simulink library "AircraftModel"  (R2016b)
settings: Solver=VariableStepAuto  StartTime=0.0  StopTime=10.0  RelTol=1e-3
values from neighbouring files (symbols this model uses):
  AC = miniMUTT_config    [UAV_config.m]
undefined symbols (not defined in the file or in its folder): Env, m, s
undefined symbols (not defined in the file): TrimCondition
libraries: aerolib6dofsys x4, Environment_Lib x2, aerolibconvert2 x2, aerolibatmos2 x1, aerolibgravity2 x1, aerolibutil x1, AuxEq_Lib x1, aerolibadyn x1, Gravity_Lib x1, Propulsion_Lib x1
settings Model: Creator=UAVLAB  LastModifiedBy=UAVLAB

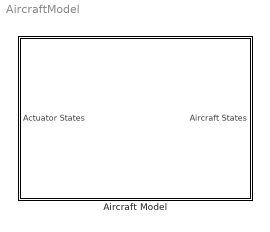
== system AircraftModel ==
  Aircraft Model : Subsystem

== system AircraftModel/Aircraft Model ==
  Actuator States : Inport  OutDataTypeStr=Bus: Actuators
  Bus Creator : BusCreator  Inputs=3  OutDataTypeStr=Bus: States
      settings: InheritFromInputs=off
  Environment Model : Subsystem
  Nonlinear UAV Model : Subsystem
  Aircraft States : Outport  OutDataTypeStr=Bus: States
  wires:
  Bus Creator/1 -> Aircraft States/1
  Environment Model/1(EnvData) -> Bus Creator/1, Nonlinear UAV Model/1(EnvData)  "EnvData"
  Nonlinear UAV Model/2(AuxVar) -> Environment Model/2(AuxVar), Bus Creator/2  "AuxVar"
  Nonlinear UAV Model/1(RigidStates) -> Bus Creator/3, Environment Model/1(RigidStates)  "RigidStates"
  Actuator States/1 -> Nonlinear UAV Model/2(Actuator States)

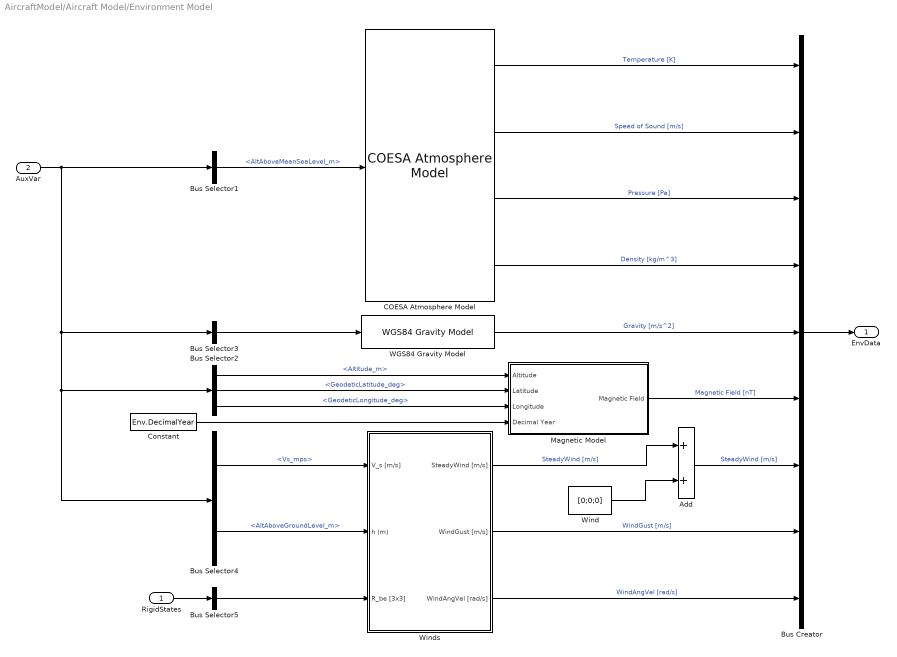
== system AircraftModel/Aircraft Model/Environment Model ==
  RigidStates : Inport  OutDataTypeStr=Bus: RigidStates
  AuxVar : Inport  Port=2  OutDataTypeStr=Bus: AuxVar
  Add : Sum
  Bus Creator : BusCreator  Inputs=9  OutDataTypeStr=Bus: EnvData
      settings: InheritFromInputs=off
  Bus Selector1 : BusSelector  OutputSignals=Nav.AltAboveMeanSeaLevel_m
  Bus Selector2 : BusSelector  OutputSignals=Nav.Altitude_m,Nav.GeodeticLatitude_deg,Nav.GeodeticLongitude_deg
  Bus Selector3 : BusSelector  OutputSignals=Nav.GeodeticLatitude_deg,Nav.GeodeticLongitude_deg,Nav.Altitude_m  OutputAsBus=on
  Bus Selector4 : BusSelector  OutputSignals=WindAxesParams.Vs_mps,Nav.AltAboveGroundLevel_m
  Bus Selector5 : BusSelector  OutputSignals=DCM  OutputAsBus=on
  COESA Atmosphere Model : aerolibatmos2/COESA Atmosphere Model  units=Metric (MKS)  spec=1976 COESA-extended U.S. Standard Atmosphere  model=Profile  profile_var=High temperature  profile_percent=1%  profile_alt=5 km (16404 ft)  envelope_var=High temperature  envelope_percent=1%  action=Warning
  Constant : Constant  Value=Env.DecimalYear
  Magnetic Model : Subsystem  BlockChoice=WMM Bypass
      settings: AttributesFormatString=%<BlockChoice>  TemplateBlock=Environment_Lib/Magnetic Model  MemberBlocks=WMM 2005,WMM Bypass
  "WGS84 Gravity Model " : aerolibgravity2/WGS84 Gravity Model   model=WGS84 Taylor Series  units=Metric (MKS)  no_atmos=on  precessing=on  jd_loc=off  month=October  day=10  year=2004  no_centrifugal=on  action=Warning
  Wind : Constant  Value=[0;0;0]
  Winds : Subsystem  BlockChoice=Wind Bypass
      settings: AttributesFormatString=%<BlockChoice>  TemplateBlock=Environment_Lib/Winds  MemberBlocks=Wind & Turbulence,Wind Bypass
  EnvData : Outport  OutDataTypeStr=Bus: EnvData
  wires:
  Winds/1(SteadyWind [m/s]) -> Add/1  "SteadyWind [m/s]"
  Wind/1 -> Add/2
  Winds/3(WindAngVel [rad/s]) -> Bus Creator/9  "WindAngVel [rad/s]"
  Winds/2(WindGust [m/s]) -> Bus Creator/8  "WindGust [m/s]"
  Add/1 -> Bus Creator/7  "SteadyWind [m/s]"
  Magnetic Model/1(Magnetic Field) -> Bus Creator/6  "Magnetic Field [nT]"
  "WGS84 Gravity Model "/1 -> Bus Creator/5  "Gravity [m/s^2]"
  Bus Selector5/1 -> Winds/3(R_be [3x3])
  RigidStates/1 -> Bus Selector5/1
  AuxVar/1 -> Bus Selector1/1, Bus Selector2/1, Bus Selector4/1, Bus Selector3/1
  Constant/1 -> Magnetic Model/4(Decimal Year)
  Bus Selector3/1 -> "WGS84 Gravity Model "/1
  Bus Selector2/3 -> Magnetic Model/3(Longitude)  "<GeodeticLongitude_deg>"
  Bus Selector2/2 -> Magnetic Model/2(Latitude)  "<GeodeticLatitude_deg>"
  Bus Selector2/1 -> Magnetic Model/1(Altitude)  "<Altitude_m>"
  COESA Atmosphere Model/4 -> Bus Creator/4  "Density [kg/m^3]"
  COESA Atmosphere Model/1 -> Bus Creator/1  "Temperature [K]"
  COESA Atmosphere Model/2 -> Bus Creator/2  "Speed of Sound [m/s]"
  COESA Atmosphere Model/3 -> Bus Creator/3  "Pressure [Pa]"
  Bus Selector1/1 -> COESA Atmosphere Model/1  "<AltAboveMeanSeaLevel_m>"
  Bus Creator/1 -> EnvData/1
  Bus Selector4/1 -> Winds/1(V_s [m/s])  "<Vs_mps>"
  Bus Selector4/2 -> Winds/2(h (m))  "<AltAboveGroundLevel_m>"

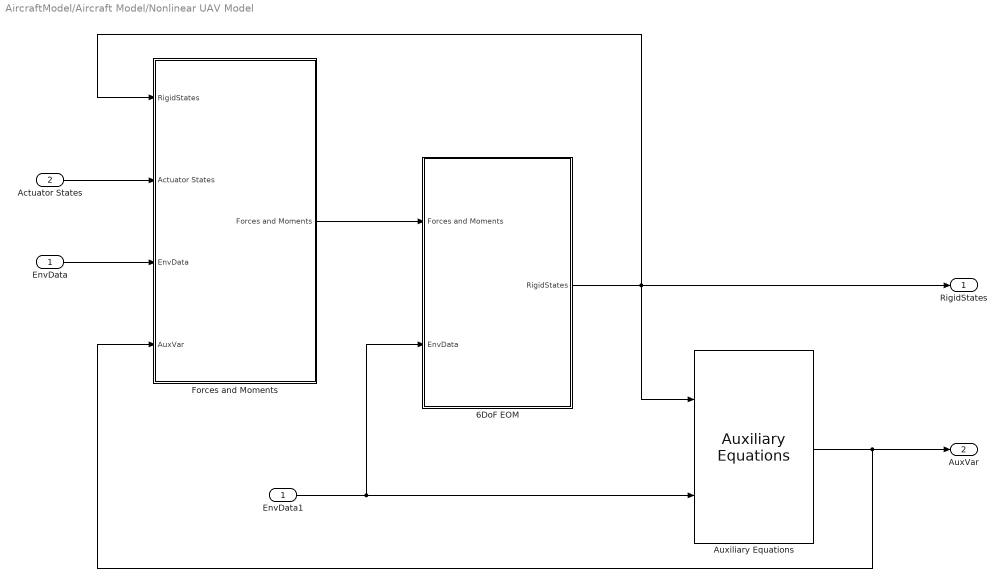
== system AircraftModel/Aircraft Model/Nonlinear UAV Model ==
  EnvData : Inport  OutDataTypeStr=Bus: EnvData
  Actuator States : Inport  Port=2  OutDataTypeStr=Bus: Actuators
  6DoF EOM : Subsystem  mask(6DoF EoM (Body Axis)){units=Metric (MKS), mtype=Fixed, rep=Euler Angles, xme_0=TrimCondition.InertialIni, Vm_0=TrimCondition.VelocitiesIni, eul_0=TrimCondition.AttitudeIni, pm_0=TrimCondition.RatesIni, mass_0=AC.Mass, mass_e=0.5, mass_f=2.0, inertia=AC.Inertia.Matrix, inertia_e=eye(3), inertia_f=2*eye(3), k_quat=1.0}
      mask prompts: mtype "Mass type:"; rep "Representation:"; xme_0 "Initial position in inertial axes [Xe,Ye,Ze]:"; Vm_0 "Initial velocity in body axes [U,v,w]:"; eul_0 "Initial Euler orientation [roll, pitch, yaw]:"; pm_0 "Initial body rotation rates [p,q,r]:"; mass_0 "Initial mass:"; mass_e "Empty mass:"; mass_f "Full mass:"; inertia_e "Empty inertia matrix:"; inertia_f "Full inertia matrix:"; k_quat "Gain for quaternion normalization:"
      mask help:
      | Integrate the six-degrees-of-freedom equations of motion in body axis.
      |
      | This block has been modified from the original Aerospace Blockset
      | implementation. The inertial position vector (Xe) is no longer computed.
      | The original block did not have a way to add steady state winds to the
      | inertial velocities (Ve) prior to integrating to get Xe. Therefore, this
      | step is performed in the Auxiliary Equations block.
      mask Help: eval('asbhelp(''sixdof_euler_angles'')');
      mask TypeOptions units: Metric (MKS) | English (Velocity in ft/s) | English (Velocity in kts)
      mask TypeOptions mtype: Fixed | Simple Variable | Custom Variable
      mask Callback mtype: aeroicon('aeroblk6dofbody');
      mask TypeOptions rep: Euler Angles | Quaternion
      mask Callback rep: aeroicon('aeroblk6dofbody');
  Auxiliary Equations : AuxEq_Lib/Auxiliary Equations
  EnvData1 : InportShadow  OutDataTypeStr=Bus: EnvData
  Forces and Moments : Subsystem
  RigidStates : Outport  OutDataTypeStr=Bus: RigidStates
  AuxVar : Outport  Port=2  OutDataTypeStr=Bus: AuxVar
  wires:
  Auxiliary Equations/1 -> AuxVar/1, Forces and Moments/4(AuxVar)
  6DoF EOM/1(RigidStates) -> Auxiliary Equations/1, RigidStates/1, Forces and Moments/1(RigidStates)
  EnvData1/1 -> Auxiliary Equations/2, 6DoF EOM/2(EnvData)
  EnvData/1 -> Forces and Moments/3(EnvData)
  Actuator States/1 -> Forces and Moments/2(Actuator States)
  Forces and Moments/1(Forces and Moments) -> 6DoF EOM/1(Forces and Moments)

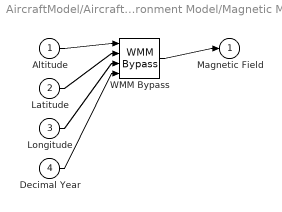
== system AircraftModel/Aircraft Model/Environment Model/Magnetic Model ==
  Altitude : Inport
  Latitude : Inport  Port=2
  Longitude : Inport  Port=3
  Decimal Year : Inport  Port=4
  WMM Bypass : Environment_Lib/WMM Bypass  units=Metric (MKS)  time_in=on  month=August  day=1  year=2009  action=None  h_out=off  dec_out=off  inc_out=off  ti_out=off
  Magnetic Field : Outport
  wires:
  WMM Bypass/1 -> Magnetic Field/1
  Decimal Year/1 -> WMM Bypass/4
  Longitude/1 -> WMM Bypass/3
  Latitude/1 -> WMM Bypass/2
  Altitude/1 -> WMM Bypass/1

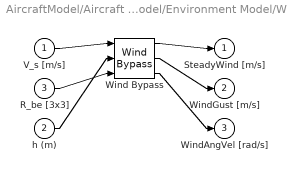
== system AircraftModel/Aircraft Model/Environment Model/Winds ==
  V_s [m/s] : Inport
  h (m) : Inport  Port=2
  R_be [3x3] : Inport  Port=3
  Wind Bypass : Environment_Lib/Wind Bypass
  SteadyWind [m/s] : Outport
  WindGust [m/s] : Outport  Port=2
  WindAngVel [rad/s] : Outport  Port=3
  wires:
  Wind Bypass/3 -> WindAngVel [rad/s]/1
  Wind Bypass/2 -> WindGust [m/s]/1
  Wind Bypass/1 -> SteadyWind [m/s]/1
  R_be [3x3]/1 -> Wind Bypass/3
  h (m)/1 -> Wind Bypass/2
  V_s [m/s]/1 -> Wind Bypass/1

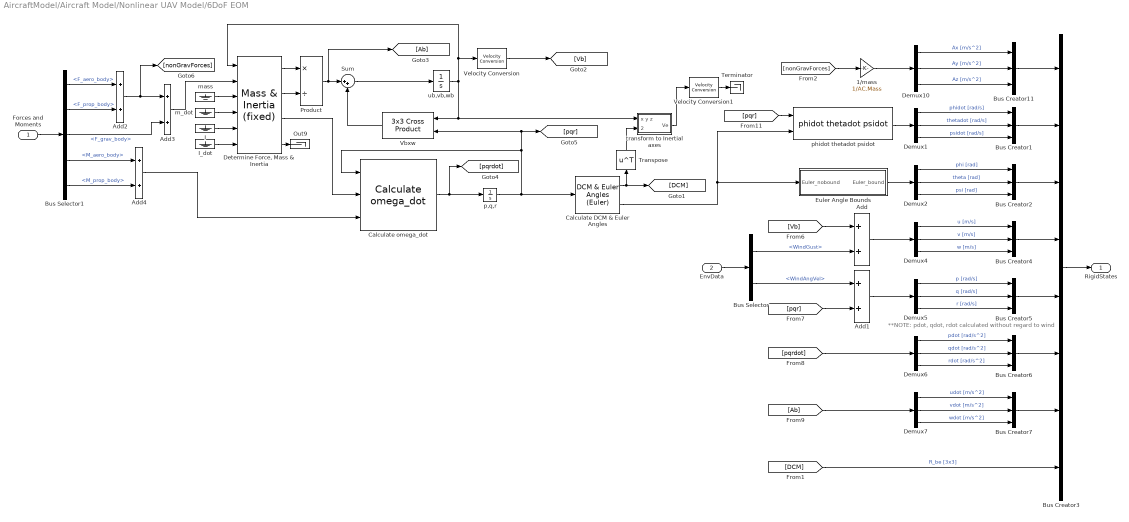
== system AircraftModel/Aircraft Model/Nonlinear UAV Model/6DoF EOM ==
  note: **NOTE: pdot, qdot, rdot calculated without regard to wind
  Forces and Moments : Inport
  EnvData : Inport  Port=2  OutDataTypeStr=Bus: EnvData
  1/mass : Gain  Gain=1/AC.Mass
  Add{,1..4} (5 alike) : Sum
  Bus Creator{1..2,4..7,11} (7 alike) : BusCreator  Inputs=3
  Bus Selector : BusSelector  OutputSignals=WindGust,WindAngVel
  Bus Selector1 : BusSelector  OutputSignals=AeroLoads.F_aero_body,F_prop_body,F_grav_body,AeroLoads.M_aero_body,M_prop_body
  Bus Creator3 : BusCreator  Inputs=8  OutDataTypeStr=Bus: RigidStates
      settings: InheritFromInputs=off
  Calculate DCM & Euler Angles : aerolib6dofsys/DCM & Euler Angles (Euler)  SystemSampleTime=-1
  Calculate omega_dot : aerolib6dofsys/Calculate omega_dot  SystemSampleTime=-1
  Demux{1..2,4..7,10} (7 alike) : Demux  Outputs=3
  "Determine Force, Mass & Inertia" : aerolib6dofsys/Mass & Inertia (fixed)  SystemSampleTime=-1
  Euler Angle Bounds : Subsystem
  I : Ground
  I_dot : Ground
  Out9 : Terminator
  Product : Product  Inputs=*/  SaturateOnIntegerOverflow=on  OutDataTypeStr=Inherit: Same as first input
  Sum : Sum  Inputs=|++  SaturateOnIntegerOverflow=on
  Terminator : Terminator
  Transpose : Math  Operator=transpose  SaturateOnIntegerOverflow=on
  Vbxw : aerolibutil/3x3 Cross Product
  Velocity Conversion : aerolibconvert2/Velocity Conversion  IU=m/s  OU=m/s
  Velocity Conversion1 : aerolibconvert2/Velocity Conversion  IU=m/s  OU=m/s
  m_dot : Ground
  mass : Ground
  "p,q,r " : Integrator  InitialCondition=pm_0
  phidot thetadot psidot : aerolib6dofsys/DCM & Euler Angles (Euler)/phidot thetadot psidot
  "transform to Inertial axes " : Subsystem  mask(Vector Transformation){}
      mask Display: disp('L_EB')
  ub,vb,wb : Integrator  InitialCondition=convvel(Vm_0,'m/s','m/s')
  RigidStates : Outport  OutDataTypeStr=Bus: RigidStates
  wires:
  [DCM] -> Bus Creator3/8  "R_be [3x3]"
  Bus Creator11/1 -> Bus Creator3/1
  Bus Creator2/1 -> Bus Creator3/3
  Bus Creator1/1 -> Bus Creator3/2
  Bus Creator7/1 -> Bus Creator3/7
  Bus Creator6/1 -> Bus Creator3/6
  Bus Creator5/1 -> Bus Creator3/5
  Bus Creator4/1 -> Bus Creator3/4
  Bus Creator3/1 -> RigidStates/1
  Add4/1 -> Calculate omega_dot/3
  Bus Selector1/5 -> Add4/2  "<M_prop_body>"
  Bus Selector1/4 -> Add4/1  "<M_aero_body>"
  Add3/1 -> "Determine Force, Mass & Inertia"/2
  Bus Selector1/3 -> Add3/2  "<F_grav_body>"
  Add2/1 -> Add3/1, [nonGravForces]
  Bus Selector1/2 -> Add2/2  "<F_prop_body>"
  Bus Selector1/1 -> Add2/1  "<F_aero_body>"
  Forces and Moments/1 -> Bus Selector1/1
  Demux10/3 -> Bus Creator11/3  "Az [m/s^2]"
  Demux10/2 -> Bus Creator11/2  "Ay [m/s^2]"
  Demux10/1 -> Bus Creator11/1  "Ax [m/s^2]"
  1/mass/1 -> Demux10/1
  [nonGravForces] -> 1/mass/1
  Euler Angle Bounds/1(Euler_bound) -> Demux2/1
  Demux2/1 -> Bus Creator2/1  "phi [rad]"
  Demux2/2 -> Bus Creator2/2  "theta [rad]"
  Demux2/3 -> Bus Creator2/3  "psi [rad]"
  Calculate DCM & Euler Angles/2 -> phidot thetadot psidot/2, Euler Angle Bounds/1(Euler_nobound)
  [pqr] -> phidot thetadot psidot/1
  phidot thetadot psidot/1 -> Demux1/1
  Demux1/1 -> Bus Creator1/1  "phidot [rad/s]"
  Demux1/2 -> Bus Creator1/2  "thetadot [rad/s]"
  Demux1/3 -> Bus Creator1/3  "psidot [rad/s]"
  Demux7/1 -> Bus Creator7/1  "udot [m/s^2]"
  Demux7/2 -> Bus Creator7/2  "vdot [m/s^2]"
  Demux7/3 -> Bus Creator7/3  "wdot [m/s^2]"
  [Ab] -> Demux7/1
  Demux6/1 -> Bus Creator6/1  "pdot [rad/s^2]"
  Demux6/2 -> Bus Creator6/2  "qdot [rad/s^2]"
  Demux6/3 -> Bus Creator6/3  "rdot [rad/s^2]"
  [pqrdot] -> Demux6/1
  Add1/1 -> Demux5/1
  Demux5/1 -> Bus Creator5/1  "p [rad/s]"
  Demux5/2 -> Bus Creator5/2  "q [rad/s]"
  Demux5/3 -> Bus Creator5/3  "r [rad/s]"
  [pqr] -> Add1/2
  Demux4/1 -> Bus Creator4/1  "u [m/s]"
  Demux4/2 -> Bus Creator4/2  "v [m/s]"
  Demux4/3 -> Bus Creator4/3  "w [m/s]"
  Add/1 -> Demux4/1
  [Vb] -> Add/1
  Bus Selector/2 -> Add1/1  "<WindAngVel>"
  Bus Selector/1 -> Add/2  "<WindGust>"
  EnvData/1 -> Bus Selector/1
  Velocity Conversion1/1 -> Terminator/1
  Velocity Conversion/1 -> [Vb]
  "Determine Force, Mass & Inertia"/3 -> Calculate omega_dot/2
  Vbxw/1 -> Sum/2
  ub,vb,wb/1 -> "transform to Inertial axes "/1(x y z), Vbxw/1, Velocity Conversion/1, "Determine Force, Mass & Inertia"/1
  Sum/1 -> ub,vb,wb/1
  "transform to Inertial axes "/1(Ve) -> Velocity Conversion1/1
  "p,q,r "/1 -> Calculate DCM & Euler Angles/1, Vbxw/2, [pqr], Calculate omega_dot/1
  Product/1 -> Sum/1, [Ab]
  Calculate DCM & Euler Angles/1 -> Transpose/1, [DCM]
  Transpose/1 -> "transform to Inertial axes "/2(transform coefficients)
  mass/1 -> "Determine Force, Mass & Inertia"/3
  "Determine Force, Mass & Inertia"/2 -> Product/2
  m_dot/1 -> "Determine Force, Mass & Inertia"/4
  "Determine Force, Mass & Inertia"/4 -> Out9/1
  Calculate omega_dot/1 -> "p,q,r "/1, [pqrdot]
  I/1 -> "Determine Force, Mass & Inertia"/5
  I_dot/1 -> "Determine Force, Mass & Inertia"/6
  "Determine Force, Mass & Inertia"/1 -> Product/1

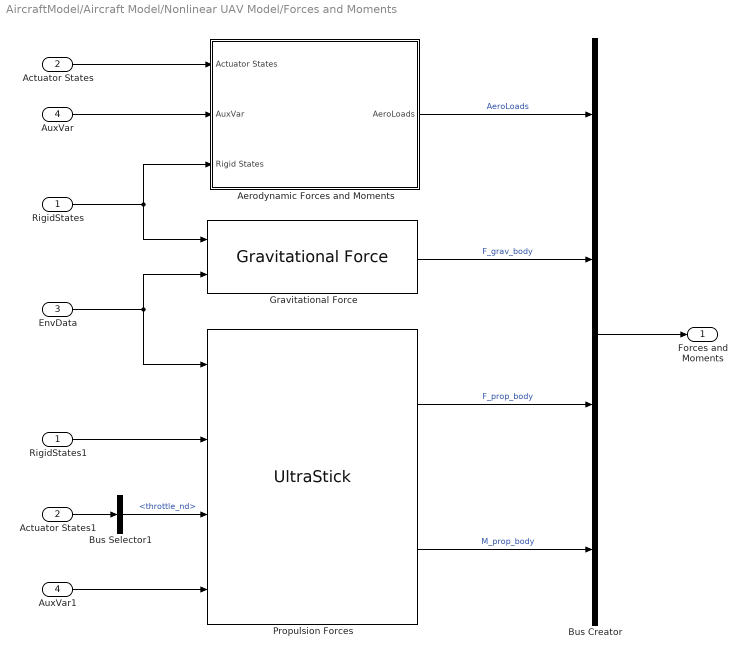
== system AircraftModel/Aircraft Model/Nonlinear UAV Model/Forces and Moments ==
  RigidStates : Inport  OutDataTypeStr=Bus: RigidStates
  Actuator States : Inport  Port=2  OutDataTypeStr=Bus: Actuators
  EnvData : Inport  Port=3  OutDataTypeStr=Bus: EnvData
  AuxVar : Inport  Port=4  OutDataTypeStr=Bus: AuxVar
  Actuator States1 : InportShadow  Port=2  OutDataTypeStr=Bus: Actuators
  Aerodynamic Forces and Moments : Subsystem
  AuxVar1 : InportShadow  Port=4  OutDataTypeStr=Bus: AuxVar
  Bus Selector1 : BusSelector  OutputSignals=throttle_nd
  Bus Creator : BusCreator  Inputs=4
  "Gravitational Force " : Gravity_Lib/Gravitational Force 
  Propulsion Forces : Propulsion_Lib/UltraStick
  RigidStates1 : InportShadow  OutDataTypeStr=Bus: RigidStates
  Forces and Moments : Outport
  wires:
  AuxVar1/1 -> Propulsion Forces/4
  RigidStates/1 -> Aerodynamic Forces and Moments/3(Rigid States), "Gravitational Force "/1
  AuxVar/1 -> Aerodynamic Forces and Moments/2(AuxVar)
  Bus Creator/1 -> Forces and Moments/1
  Propulsion Forces/2 -> Bus Creator/4  "M_prop_body"
  Propulsion Forces/1 -> Bus Creator/3  "F_prop_body"
  "Gravitational Force "/1 -> Bus Creator/2  "F_grav_body"
  RigidStates1/1 -> Propulsion Forces/2
  Aerodynamic Forces and Moments/1(AeroLoads) -> Bus Creator/1  "AeroLoads"
  Bus Selector1/1 -> Propulsion Forces/3  "<throttle_nd>"
  EnvData/1 -> "Gravitational Force "/2, Propulsion Forces/1
  Actuator States1/1 -> Bus Selector1/1
  Actuator States/1 -> Aerodynamic Forces and Moments/1(Actuator States)

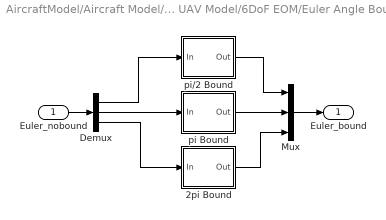
== system AircraftModel/Aircraft Model/Nonlinear UAV Model/6DoF EOM/Euler Angle Bounds ==
  Euler_nobound : Inport
  2pi Bound : Subsystem
  Demux : Demux  Outputs=3
  Mux : Mux  Inputs=3
  pi Bound : Subsystem
  pi/2 Bound : Subsystem
  Euler_bound : Outport
  wires:
  2pi Bound/1(Out) -> Mux/3
  Demux/3 -> 2pi Bound/1(In)
  Demux/2 -> pi Bound/1(In)
  Demux/1 -> pi/2 Bound/1(In)
  Euler_nobound/1 -> Demux/1
  Mux/1 -> Euler_bound/1
  pi/2 Bound/1(Out) -> Mux/1
  pi Bound/1(Out) -> Mux/2

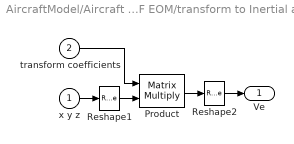
== system AircraftModel/Aircraft Model/Nonlinear UAV Model/6DoF EOM/transform to Inertial axes  ==
  x y z : Inport
  transform coefficients : Inport  Port=2
  Product : Product  Multiplication=Matrix(*)  SaturateOnIntegerOverflow=on  InputSameDT=on  OutDataTypeStr=Inherit: Same as first input
  Reshape1 : Reshape  OutputDimensionality=Column vector (2-D)
  Reshape2 : Reshape
  Ve : Outport
  wires:
  Product/1 -> Reshape2/1
  transform coefficients/1 -> Product/1
  x y z/1 -> Reshape1/1
  Reshape1/1 -> Product/2
  Reshape2/1 -> Ve/1

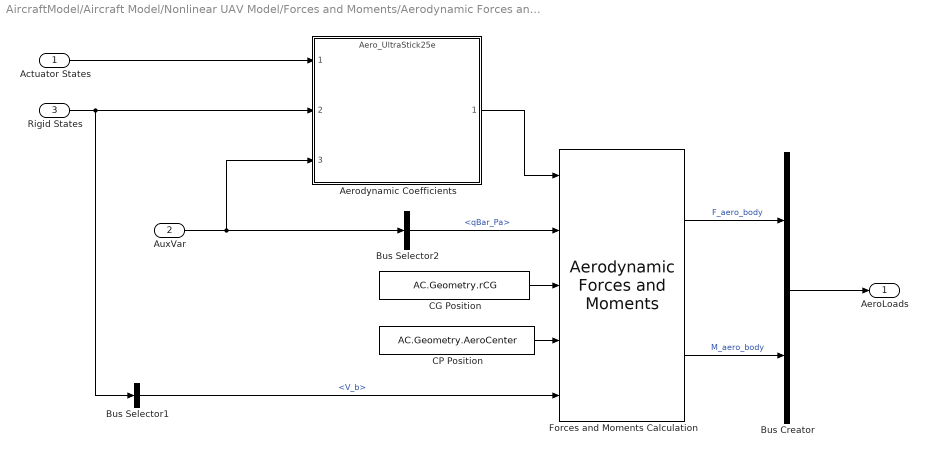
== system AircraftModel/Aircraft Model/Nonlinear UAV Model/Forces and Moments/Aerodynamic Forces and Moments ==
  Actuator States : Inport  OutDataTypeStr=Bus: Actuators
  AuxVar : Inport  Port=2
  Rigid States : Inport  Port=3  OutDataTypeStr=Bus: RigidStates
  Aerodynamic Coefficients : ModelReference  ModelNameDialog=Aero_UltraStick25e  SimulationMode=Normal  Variant=on  ModelReferenceVersion=1.2
  Bus Selector1 : BusSelector  OutputSignals=V_b
  Bus Creator : BusCreator  Inputs=2
  Bus Selector2 : BusSelector  OutputSignals=qBar_Pa
  CG Position : Constant  Value=AC.Geometry.rCG
  CP Position : Constant  Value=AC.Geometry.AeroCenter
  Forces and Moments Calculation : aerolibadyn/Aerodynamic Forces and Moments   inputAxes=Wind  outputForceAxes=Body  outputMomentAxes=Wind  S=AC.Geometry.S  b=AC.Geometry.b  cbar=AC.Geometry.c
  AeroLoads : Outport
  wires:
  Actuator States/1 -> Aerodynamic Coefficients/1
  Aerodynamic Coefficients/1 -> Forces and Moments Calculation/1
  Bus Selector2/1 -> Forces and Moments Calculation/2  "<qBar_Pa>"
  AuxVar/1 -> Bus Selector2/1, Aerodynamic Coefficients/3
  Forces and Moments Calculation/2 -> Bus Creator/2  "M_aero_body"
  Bus Creator/1 -> AeroLoads/1
  Forces and Moments Calculation/1 -> Bus Creator/1  "F_aero_body"
  Rigid States/1 -> Aerodynamic Coefficients/2, Bus Selector1/1
  CP Position/1 -> Forces and Moments Calculation/4
  CG Position/1 -> Forces and Moments Calculation/3
  Bus Selector1/1 -> Forces and Moments Calculation/5  "<V_b>"

== system AircraftModel/Aircraft Model/Nonlinear UAV Model/6DoF EOM/Euler Angle Bounds/2pi Bound ==
  In : Inport
  2pi : Constant  Value=2*pi
  Math Function2 : Math  Operator=mod  SaturateOnIntegerOverflow=on
  Out : Outport
  wires:
  In/1 -> Math Function2/1
  2pi/1 -> Math Function2/2
  Math Function2/1 -> Out/1

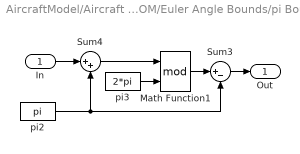
== system AircraftModel/Aircraft Model/Nonlinear UAV Model/6DoF EOM/Euler Angle Bounds/pi Bound ==
  In : Inport
  Math Function1 : Math  Operator=mod  SaturateOnIntegerOverflow=on
  Sum3 : Sum  Inputs=|+-  SaturateOnIntegerOverflow=on  InputSameDT=on  OutDataTypeStr=Inherit: Same as first input
  Sum4 : Sum  Inputs=|++  SaturateOnIntegerOverflow=on  InputSameDT=on  OutDataTypeStr=Inherit: Same as first input
  pi2 : Constant  Value=pi
  pi3 : Constant  Value=2*pi
  Out : Outport
  wires:
  Sum3/1 -> Out/1
  pi2/1 -> Sum3/2, Sum4/2
  Sum4/1 -> Math Function1/1
  In/1 -> Sum4/1
  pi3/1 -> Math Function1/2
  Math Function1/1 -> Sum3/1

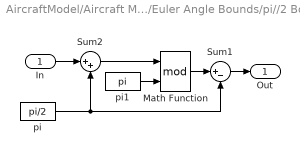
== system AircraftModel/Aircraft Model/Nonlinear UAV Model/6DoF EOM/Euler Angle Bounds/pi//2 Bound ==
  In : Inport
  Math Function : Math  Operator=mod  SaturateOnIntegerOverflow=on
  Sum1 : Sum  Inputs=|+-  SaturateOnIntegerOverflow=on  InputSameDT=on  OutDataTypeStr=Inherit: Same as first input
  Sum2 : Sum  Inputs=|++  SaturateOnIntegerOverflow=on  InputSameDT=on  OutDataTypeStr=Inherit: Same as first input
  pi : Constant  Value=pi/2
  pi1 : Constant  Value=pi
  Out : Outport
  wires:
  Math Function/1 -> Sum1/1
  pi1/1 -> Math Function/2
  In/1 -> Sum2/1
  Sum2/1 -> Math Function/1
  pi/1 -> Sum2/2, Sum1/2
  Sum1/1 -> Out/1
